simulink model "m_modelcov02"  (Simulink 7.8)
settings: Solver=FixedStepDiscrete  StartTime=0.0  StopTime=1  FixedStep=0.1  RelTol=1e-3
Description:
  | Cruise Control Test Generation
settings Model: Creator=The MathWorks Inc.  LastModifiedBy=itoy  RecordCoverage=on  CovMetricSettings=dcms  CovHTMLOptions=-aTS=1 -bRG=1 -bTC=1 -hTR=0 -nFC=0 -scm=1 -bcm=1 -xEv=0  covSaveCumulativeToWorkspaceVar=off  CovSaveSingleToWorkspaceVar=off
settings DataIOCC: LimitDataPoints=off  SaveFormat=StructureWithTime  SaveOutput=off  SaveTime=off
settings OptimizationCC: ConditionallyExecuteInputs=off  InlineParams=on  InlineInvariantSignals=on  InitFltsAndDblsToZero=on  EfficientMapNaN2IntZero=off
settings DebuggingCC: SaveWithParameterizedLinksMsg=none  SignalResolutionControl=TryResolveAllWithWarning  FcnCallInpInsideContextMsg=Use local settings  StrictBusMsg=Warning
settings GRTTargetCC: TargetFcnLib=ansi_tfl_tmw.mat
settings ConfigComp: Description=Design Verifier Custom Configuration Component  DVMaxProcessTime=60  DVMakeOutputFilesUnique=off  DVParameters=on  DVModelCoverageObjectives=MCDC  DVMaxTestCaseSteps=500  DVTestSuiteOptimization=CombinedObjectives  DVAssertions=EnableAll  DVProofAssumptions=EnableAll  DVProvingStrategy=FindViolation

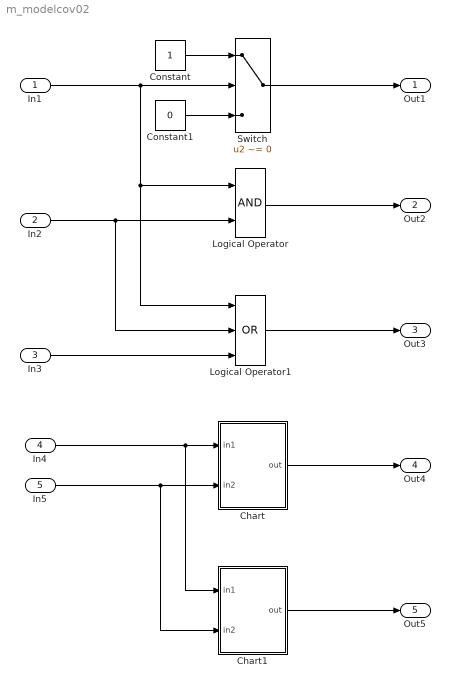
== system m_modelcov02 ==
  In1 : Inport
  In2 : Inport  Port=2
  In3 : Inport  Port=3
  In4 : Inport  Port=4
  In5 : Inport  Port=5
  Chart : Stateflow chart  TreatAsAtomicUnit=on
  Chart1 : Stateflow chart  TreatAsAtomicUnit=on
  Constant : Constant
  Constant1 : Constant  Value=0
  Logical Operator : Logic  AllPortsSameDT=off  OutDataTypeStr=boolean
  Logical Operator1 : Logic  Operator=OR  Inputs=3  AllPortsSameDT=off  OutDataTypeStr=boolean
  Switch : Switch  Criteria=u2 ~= 0
  Out1 : Outport
  Out2 : Outport  Port=2
  Out3 : Outport  Port=3
  Out4 : Outport  Port=4
  Out5 : Outport  Port=5
  wires:
  Constant/1 -> Switch/1
  In1/1 -> Switch/2, Logical Operator1/1, Logical Operator/1
  Constant1/1 -> Switch/3
  Switch/1 -> Out1/1
  In2/1 -> Logical Operator/2, Logical Operator1/2
  In3/1 -> Logical Operator1/3
  Logical Operator/1 -> Out2/1
  Logical Operator1/1 -> Out3/1
  In4/1 -> Chart/1(in1), Chart1/1(in1)
  In5/1 -> Chart/2(in2), Chart1/2(in2)
  Chart/1(out) -> Out4/1
  Chart1/1(out) -> Out5/1

== stateflow chart Chart ==
  state P/
    state A/
      out = 1;
    state B/
      out = 0;
    (default) -> A
    A -> B : [ in1 == 0 ]
    B -> A : [ in1 ~= 0 ]
  state C/
    out = 2;
  (default) -> P
  P -> C : [in2 == 1]
  C -> A : [in2 ~= 1]
  data: in1 input double; in2 input double; out output uint8

== stateflow chart Chart1 ==
  (default) -> (junction 18)
  (junction 18) -> (junction 19) [order 2] : {
      | out = 1;
      | }
  (junction 18) -> (junction 20) [order 1] : [ in1 == 1 && in2 == 0 ]
  (junction 20) -> (junction 21) : {
      | out = 0;
      | }
  data: in1 input double; in2 input double; out output uint8
